simulink model "dpd_top_fixed"  (R2025b)
settings: Solver=FixedStepDiscrete  StartTime=0.0  StopTime=length(tx_bb)*Ts  FixedStep=Ts  RelTol=1e-3
undefined symbols (not defined in the file): Ts
settings Model: Creator=zhuyong  LastModifiedBy=zhuyong

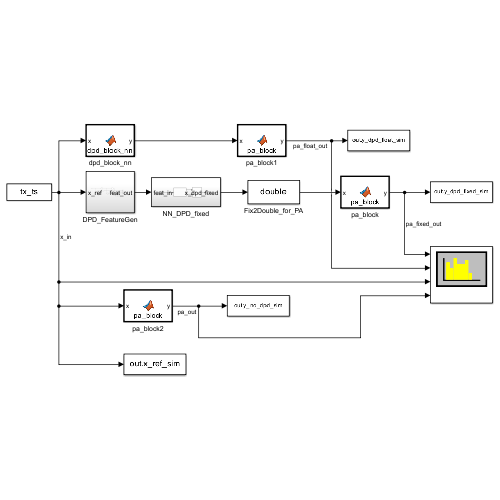
[thumbnail: Simulink's stored preview of the top-level diagram]
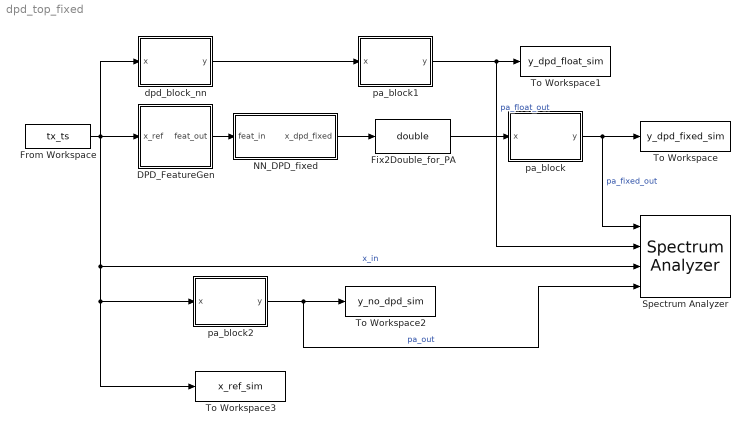
== system dpd_top_fixed ==
  DPD_FeatureGen : Subsystem
  Fix2Double_for_PA : DataTypeConversion  OutDataTypeStr=double  SaturateOnIntegerOverflow=off  RndMeth=Floor
  From Workspace : FromWorkspace  VariableName=tx_ts  SampleTime=Ts
  NN_DPD_fixed : Subsystem
  Spectrum Analyzer : SpectrumAnalyzer  NumInputPorts=4  WindowPosition=[1.000000,49.000000,1536.000000,793.000000,]  ScopeFrameLocation=window  SampleRateSource=Property  SampleRate=Fs  WindowInvariantSamplesPerUpdate=on  Span=122880000  StartFrequency=-61440000  StopFrequency=61440000  MaximizeAxes=Off  YLimits=[22.8933 29.6078]  ShowLegend=on
  To Workspace : ToWorkspace  VariableName=y_dpd_fixed_sim  SampleTime=Ts
  To Workspace1 : ToWorkspace  VariableName=y_dpd_float_sim  SampleTime=Ts
  To Workspace2 : ToWorkspace  VariableName=y_no_dpd_sim  SampleTime=Ts
  To Workspace3 : ToWorkspace  VariableName=x_ref_sim  SampleTime=Ts
  dpd_block_nn : MATLAB Function  TreatAsAtomicUnit=on
  pa_block : MATLAB Function  TreatAsAtomicUnit=on
  pa_block1 : MATLAB Function  TreatAsAtomicUnit=on
  pa_block2 : MATLAB Function  TreatAsAtomicUnit=on
  wires:
  From Workspace/1 -> To Workspace3/1, pa_block2/1(x), Spectrum Analyzer/3, dpd_block_nn/1(x), DPD_FeatureGen/1(x_ref)  "x_in"
  pa_block/1(y) -> To Workspace/1, Spectrum Analyzer/1  "pa_fixed_out"
  DPD_FeatureGen/1(feat_out) -> NN_DPD_fixed/1(feat_in)
  NN_DPD_fixed/1(x_dpd_fixed) -> Fix2Double_for_PA/1
  pa_block1/1(y) -> To Workspace1/1, Spectrum Analyzer/2  "pa_float_out"
  dpd_block_nn/1(y) -> pa_block1/1(x)
  Fix2Double_for_PA/1 -> pa_block/1(x)
  pa_block2/1(y) -> Spectrum Analyzer/4, To Workspace2/1  "pa_out"

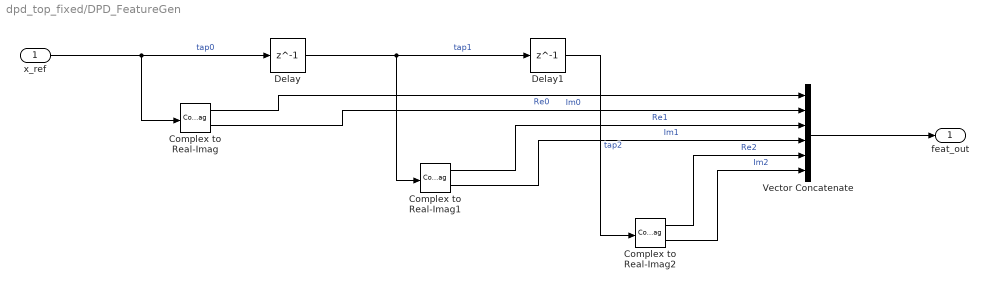
== system dpd_top_fixed/DPD_FeatureGen ==
  x_ref : Inport
  Complex to Real-Imag : ComplexToRealImag
  Complex to Real-Imag1 : ComplexToRealImag
  Complex to Real-Imag2 : ComplexToRealImag
  Delay : Delay  DelayLength=1  SampleTime=Ts
  Delay1 : Delay  DelayLength=1  SampleTime=Ts
  Vector Concatenate : Concatenate  NumInputs=6
  feat_out : Outport
  wires:
  x_ref/1 -> Complex to Real-Imag/1, Delay/1  "tap0"
  Delay/1 -> Delay1/1, Complex to Real-Imag1/1  "tap1"
  Delay1/1 -> Complex to Real-Imag2/1  "tap2"
  Complex to Real-Imag/1 -> Vector Concatenate/1  "Re0"
  Complex to Real-Imag/2 -> Vector Concatenate/2  "Im0"
  Complex to Real-Imag1/1 -> Vector Concatenate/3  "Re1"
  Complex to Real-Imag1/2 -> Vector Concatenate/4  "Im1"
  Complex to Real-Imag2/1 -> Vector Concatenate/5  "Re2"
  Complex to Real-Imag2/2 -> Vector Concatenate/6  "Im2"
  Vector Concatenate/1 -> feat_out/1

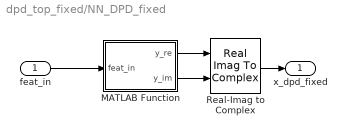
== system dpd_top_fixed/NN_DPD_fixed ==
  feat_in : Inport
  MATLAB Function : MATLAB Function  TreatAsAtomicUnit=on
  Real-Imag to Complex : RealImagToComplex
  x_dpd_fixed : Outport
  wires:
  feat_in/1 -> MATLAB Function/1(feat_in)
  Real-Imag to Complex/1 -> x_dpd_fixed/1
  MATLAB Function/1(y_re) -> Real-Imag to Complex/1
  MATLAB Function/2(y_im) -> Real-Imag to Complex/2

== matlab function dpd_top_fixed/pa_block ==
  data: x input double size=[1 1]; y output double size=[1 1]
function y = pa_block(x)
%#codegen
% 在线记忆多项式 PA 模型（与 pa_memory_poly 一致的形式）
% x、y：标量复数输入输出（逐样本处理）

persistent buf;
if isempty(buf)
    buf = complex(zeros(3,1));   % K = 3 tap 记忆
end

% 更新 buffer：buf(1) 保存当前样本，buf(2)、buf(3) 为过去样本
buf = [x; buf(1:end-1)];

% 系数（与 pa_memory_poly 中保持一致或相近）
a11 = 1.0;   a12 = -0.05;  a13 = 0.02;   % 1 阶
a31 = 0.8;   a32 = -0.04;  a33 = 0.015;  % 3 阶
a51 = 0.3;   a52 = -0.02;  a53 = 0.010;  % 5 阶

acc = complex(0,0);
for k = 1:3
    xnk = buf(k);
    r   = abs(xnk);
    acc = acc ...
        + eval1(a11,a12,a13,k) * xnk ...
        + eval1(a31,a32,a33,k) * xnk * (r^2) ...
        + eval1(a51,a52,a53,k) * xnk * (r^4);
end

y = acc;

% 内部小函数：根据 tap 选择对应的系数
function c = eval1(c1,c2,c3,idx)
    if idx == 1
        c = c1;
    elseif idx == 2
        c = c2;
    else
        c = c3;
    end
end

end

== matlab function dpd_top_fixed/dpd_block_nn ==
  data: x input; y output
function y = dpd_block_nn(x)
%#codegen
% dpd_block_nn  基于已训练 NN 的预失真器（仿真专用）
%
% 输入：
%   x : 当前时刻的理想基带输入（complex double 标量）
% 输出：
%   y : 送入 PA 的预失真输出（complex double 标量）

% 声明外部预测函数为 extrinsic（只在仿真中由 MATLAB 执行）
coder.extrinsic('nn_dpd_predict');

% 记忆阶数（与训练时的 K 一致，这里直接写死）
K = 3;

% 持久化记忆 buffer（K×1 复数）
persistent buf
if isempty(buf)
    buf = complex(zeros(K,1));
end

% 确保 x 为 complex double
x = complex(x);

% 更新记忆：buf(1) = x[n], buf(2..K) = x[n-1..n-K+1]
buf = [x; buf(1:end-1)];

% 构造特征向量 feat: 1×(2K)
feat = zeros(1, 2*K);   % double
for k = 1:K
    feat(2*k-1) = real(buf(k));
    feat(2*k)   = imag(buf(k));
end

% 预分配 y_pred，显式告诉代码生成：这是 1×2 double
y_pred = zeros(1,2);
% 调用外部 NN 预测函数
y_pred = nn_dpd_predict(feat);   % extrinsic 调用

% 组合为复数输出
y = complex(y_pred(1), y_pred(2));

end

== matlab function dpd_top_fixed/pa_block1 ==
  data: x input; y output
function y = pa_block(x)
%#codegen
% 在线记忆多项式 PA 模型（与 pa_memory_poly 一致的形式）
% x、y：标量复数输入输出（逐样本处理）

persistent buf;
if isempty(buf)
    buf = complex(zeros(3,1));   % K = 3 tap 记忆
end

% 更新 buffer：buf(1) 保存当前样本，buf(2)、buf(3) 为过去样本
buf = [x; buf(1:end-1)];

% 系数（与 pa_memory_poly 中保持一致或相近）
a11 = 1.0;   a12 = -0.05;  a13 = 0.02;   % 1 阶
a31 = 0.8;   a32 = -0.04;  a33 = 0.015;  % 3 阶
a51 = 0.3;   a52 = -0.02;  a53 = 0.010;  % 5 阶

acc = complex(0,0);
for k = 1:3
    xnk = buf(k);
    r   = abs(xnk);
    acc = acc ...
        + eval1(a11,a12,a13,k) * xnk ...
        + eval1(a31,a32,a33,k) * xnk * (r^2) ...
        + eval1(a51,a52,a53,k) * xnk * (r^4);
end

y = acc;

% 内部小函数：根据 tap 选择对应的系数
function c = eval1(c1,c2,c3,idx)
    if idx == 1
        c = c1;
    elseif idx == 2
        c = c2;
    else
        c = c3;
    end
end

end

== matlab function dpd_top_fixed/pa_block2 ==
  data: x input; y output
function y = pa_block(x)
%#codegen
% 在线记忆多项式 PA 模型（与 pa_memory_poly 一致的形式）
% x、y：标量复数输入输出（逐样本处理）

persistent buf;
if isempty(buf)
    buf = complex(zeros(3,1));   % K = 3 tap 记忆
end

% 更新 buffer：buf(1) 保存当前样本，buf(2)、buf(3) 为过去样本
buf = [x; buf(1:end-1)];

% 系数（与 pa_memory_poly 中保持一致或相近）
a11 = 1.0;   a12 = -0.05;  a13 = 0.02;   % 1 阶
a31 = 0.8;   a32 = -0.04;  a33 = 0.015;  % 3 阶
a51 = 0.3;   a52 = -0.02;  a53 = 0.010;  % 5 阶

acc = complex(0,0);
for k = 1:3
    xnk = buf(k);
    r   = abs(xnk);
    acc = acc ...
        + eval1(a11,a12,a13,k) * xnk ...
        + eval1(a31,a32,a33,k) * xnk * (r^2) ...
        + eval1(a51,a52,a53,k) * xnk * (r^4);
end

y = acc;

% 内部小函数：根据 tap 选择对应的系数
function c = eval1(c1,c2,c3,idx)
    if idx == 1
        c = c1;
    elseif idx == 2
        c = c2;
    else
        c = c3;
    end
end

end

== matlab function dpd_top_fixed/NN_DPD_fixed/MATLAB Function ==
  data: feat_in input double size=[6 1]; y_re output fixdt(1,12,11) size=[1 1]; y_im output fixdt(1,12,11) size=[1 1]
function [y_re, y_im] = NN_DPD_core_fixed(feat_in)
%#codegen
% feat_in: [6x1] 实数向量（[Re0;Im0;Re1;Im1;Re2;Im2]）
% y_re, y_im: 输出的 NN-DPD 实部、虚部（定点）

    % ================== 0. 固定常量设置 ==================
    % 当前网络 K=3（3 个记忆抽头，对应 6 维特征）
    K  = 3;
    WL = 12;   % 定点总位宽（和你选择的 B_A 对齐）
    FL = 11;   % 小数位（通常取 WL-1，幅度约 [-1,1)）

    % 统一的 fimath：强制乘法 / 求和结果仍然是 (WL, FL)
    F = fimath( ...
        'RoundingMethod',      'Nearest', ...
        'OverflowAction',      'Saturate', ...
        'ProductMode',         'SpecifyPrecision', ...
        'ProductWordLength',   WL, ...
        'ProductFractionLength', FL, ...
        'SumMode',             'SpecifyPrecision', ...
        'SumWordLength',       WL, ...
        'SumFractionLength',   FL);

    % ================== 1. persistent + coder.load ==================
    % 注意：从 mat 中读取的 fi 先转成 double 保存，
    % 真正运算时再用统一的 (WL,FL,F) 转成 fi，避免类型冲突

    persistent W1d b1d W2d b2d W3d b3d

    if isempty(W1d)
        S = coder.load('../hdl/nn_dpd_fixed_params.mat', ...
                       'W1_fi','b1_fi','W2_fi','b2_fi','W3_fi','b3_fi');

        % 量化后的权重 / 偏置 -> double 常量
        W1d = double(S.W1_fi);   % [N1 x 2K]
        b1d = double(S.b1_fi);   % [N1 x 1]
        W2d = double(S.W2_fi);   % [N2 x N1]
        b2d = double(S.b2_fi);
        W3d = double(S.W3_fi);   % [2 x N2]
        b3d = double(S.b3_fi);
    end

    % ================== 2. 输入向量 -> 统一定点向量 ==================
    % feat_in 在端口属性里声明为 [6x1] double
    feat_vec = feat_in(:);                                   % 强制列向量
    feat     = fi(feat_vec, 1, WL, FL, F);                   % sfix12_En11

    % ================== 3. 第一层：fc1 + ReLU ==================
    N1 = size(W1d, 1);    % 隐层神经元数，例如 64

    a1 = fi(zeros(N1,1), 1, WL, FL, F);                      % sfix12_En11
    for i = 1:N1
        acc = fi(0, 1, WL, FL, F);                           % sfix12_En11
        % 2*K = 6，为编译期常量
        for j = 1:(2*K)
            w_ij = fi(W1d(i,j), 1, WL, FL, F);               % sfix12_En11
            % 在 fimath F 作用下：w_ij * feat(j) 结果仍为 (WL,FL)
            acc  = acc + w_ij * feat(j);                     % 不会再长成 sfix25
        end
        b_i = fi(b1d(i), 1, WL, FL, F);
        acc = acc + b_i;

        % ReLU
        if acc < 0
            a1(i) = fi(0, 1, WL, FL, F);
        else
            a1(i) = acc;
        end
    end

    % ================== 4. 第二层：fc2 + ReLU ==================
    N2 = size(W2d, 1);    % 第二层神经元数

    a2 = fi(zeros(N2,1), 1, WL, FL, F);
    for i = 1:N2
        acc = fi(0, 1, WL, FL, F);
        for j = 1:N1
            w_ij = fi(W2d(i,j), 1, WL, FL, F);
            acc  = acc + w_ij * a1(j);                       % 类型仍 (WL,FL)
        end
        b_i = fi(b2d(i), 1, WL, FL, F);
        acc = acc + b_i;

        if acc < 0
            a2(i) = fi(0, 1, WL, FL, F);
        else
            a2(i) = acc;
        end
    end

    % ================== 5. 输出层：fc_out（2 维：Re, Im） ==================
    z_out = fi(zeros(2,1), 1, WL, FL, F);
    for i = 1:2
        acc = fi(0, 1, WL, FL, F);
        for j = 1:N2
            w_ij = fi(W3d(i,j), 1, WL, FL, F);
            acc  = acc + w_ij * a2(j);
        end
        b_i    = fi(b3d(i), 1, WL, FL, F);
        acc    = acc + b_i;
        z_out(i) = acc;
    end

    % ================== 6. 输出给 Complex 块 ==================
    y_re = z_out(1);    % sfix12_En11
    y_im = z_out(2);
end
